simulink subsystem "FuncEncoder"  (R2023b)
settings: Solver=VariableStepAuto  StartTime=0.0  StopTime=10.0  RelTol=1e-3
libraries: simulink x1
settings Model: Creator=Claudia Ada  LastModifiedBy=pablo

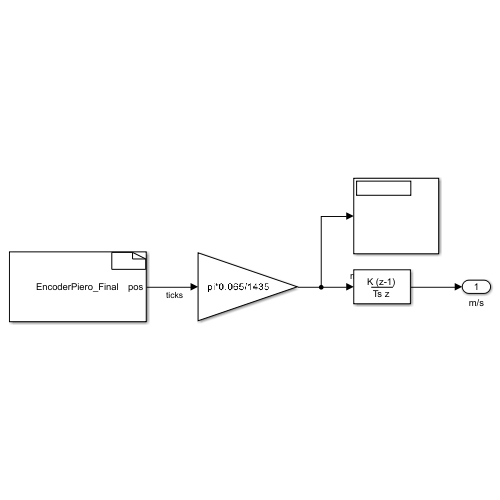
[thumbnail: Simulink's stored preview of the top-level diagram]
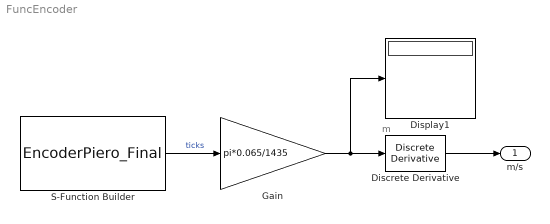
== system FuncEncoder ==
  note: m
  Discrete Derivative : simulink/Discrete/Discrete Derivative  gainval=1.0  ICPrevScaledInput=0.0  OutMin=[]  OutMax=[]  OutDataType=fixdt(1, 16)  OutScaling=2^-10  DoSatur=off
  Display1 : Display
  Gain : Gain  Gain=pi*0.065/1435  OutDataTypeStr=double
  S-Function Builder : S-Function  FunctionName=EncoderPiero_Final  SFunctionModules=EncoderPiero_Final_wrapper  SFunctionDeploymentMode=off  EnableBusSupport=off  mask(S-Function Builder){}
      mask help: Simulink:masks:SFunctionBuilder_MD
      mask init:
      | val = [[.9  0.75 0.75 1 1 .9 .9 1]',[1 1 0.75 0.75 .9 .9 1 .9]'];try , sys = get_param(gcb,'SfunBuilderFcnName');if isempty(sys), sys = get_param(gcb,'FunctionName'); end,catch, sys = get_param(gcb,'FunctionName'); end
      settings: CopyFcn=set_param(gcbh,'LinkStatus','none')  OpenFcn=sfunctionwizard(gcbh)
      mask Display: plot(val(:,1),val(:,2)),disp(sys),port_label('output',1,'pos')
  m/s : Outport
  wires:
  Discrete Derivative/1 -> m/s/1
  S-Function Builder/1 -> Gain/1  "ticks"
  Gain/1 -> Discrete Derivative/1, Display1/1
